simulink model "dsp_project"  (R2024b)
settings: Solver=VariableStepAuto  StartTime=0.0  StopTime=50  RelTol=1e-3
values from neighbouring files (symbols this model uses):
  Lf = max(1, round(freq_mask_smooth_hz / (fs/nfft)))    [dsp_project_matalb.m]    (also in dsp_project_nonstaion.m)
  Lt = max(1, round(time_mask_smooth_ms / (hop/fs*1e3)))    [dsp_project_matalb.m]    (also in dsp_project_nonstaion.m)
  n_std_thresh = 1.2    [dsp_project_matalb.m]    (also in dsp_project_nonstaion.m = 1.5)
libraries: dspvision x3, dspxfrm3 x2, dspstat3 x2, dspsigops x1
settings Model: Creator=settlab  LastModifiedBy=settlab

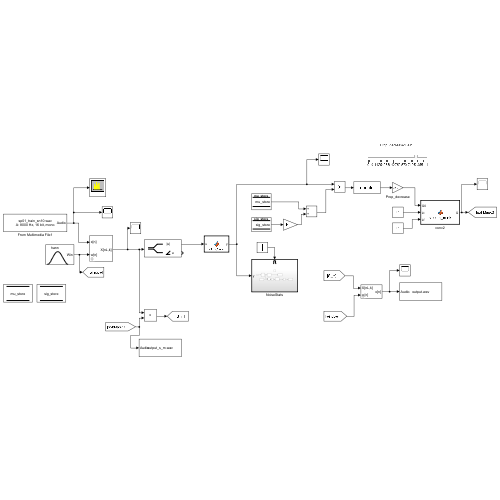
[thumbnail: Simulink's stored preview of the top-level diagram]
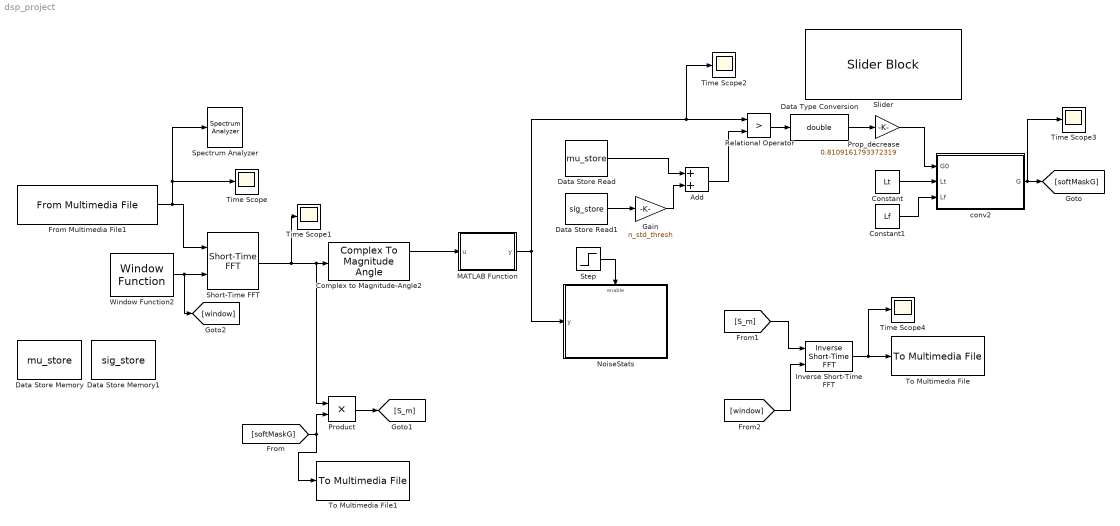
== system dsp_project ==
  Add : Sum
  Complex to Magnitude-Angle2 : ComplexToMagnitudeAngle
  Constant : Constant  Value=Lt
  Constant1 : Constant  Value=Lf
  Data Store Memory : DataStoreMemory  DataStoreName=mu_store  WriteAfterWriteMsg=warning  InitialValue=zeros(1024,1)  VectorParams1D=off  ShowAdditionalParam=off  OutDataTypeStr=double
  Data Store Memory1 : DataStoreMemory  DataStoreName=sig_store  WriteAfterWriteMsg=warning  InitialValue=zeros(1024,1)  VectorParams1D=off  ShowAdditionalParam=off  OutDataTypeStr=double
  Data Store Read : DataStoreRead  DataStoreName=mu_store  DataStoreElements=mu_store  EnableIndexing=on  NumberOfDimensions=2  IndexOptions=Index vector (dialog),Index vector (dialog)  Indices=1,1  OutputSizes=1,1
  Data Store Read1 : DataStoreRead  DataStoreName=sig_store  DataStoreElements=sig_store  EnableIndexing=on  NumberOfDimensions=2  IndexOptions=Index vector (dialog),Index vector (dialog)  Indices=1,1  OutputSizes=1,1
  Data Type Conversion : DataTypeConversion  OutDataTypeStr=double  SaturateOnIntegerOverflow=off  RndMeth=Floor
  From Multimedia File1 : dspvision/From Multimedia File  inputFilename=C:\Users\settlab\Downloads\sp01_train_sn10.wav  readRange=[1 Inf]  loop=on  numPlays=inf  outputStreams=오디오 전용  videoDataType=single  audioDataType=double  inheritSampleTime=on  userDefinedSampleTime=fs  noAudioOutput=off  isIntensityVideo=off  fourcc=RGB  colorVideoFormat=One multidimensional signal  outputEOF=off  dataOrg=Column-major  audioFrameSize=1024  computeAudioFrameSize=off  outSamplingMode=Sample based
      settings: LibrarySourceBlock=dspsrcs4/From Multimedia File
  Gain : Gain  Gain=n_std_thresh
  Inverse Short-Time FFT : dspxfrm3/Inverse  Short-Time FFT  W=1024  OvLap=768  OutFrameSize=256  InConjSymm=on  DoAssert=on  Tol=1e-4  OutputFrames=off
  MATLAB Function : MATLAB Function  TreatAsAtomicUnit=on
  NoiseStats : Subsystem  TreatAsAtomicUnit=on
  Product : Product
  Prop_decrease : Gain  Gain=0.8109161793372319  RndMeth=Nearest
  Relational Operator : RelationalOperator  Operator=>  OutDataTypeStr=boolean  ZeroCross=off  InputSameDT=off
  Short-Time FFT : dspxfrm3/Short-Time FFT  W=1024  OvLap=768  M=1024
  Slider : SliderBlock  ScaleMax=1
  Spectrum Analyzer : SpectrumAnalyzer  WindowPosition=[371.000000,449.000000,800.000000,572.000000,]  Visible=on  ScopeFrameLocation=window  ViewType=Spectrum and spectrogram  Method=Welch  PlotAsTwoSidedSpectrum=off  AveragingMethod=Exponential  YLimits=[-106.52525462,-0.29681245]  ColorLimits=[-106.52525462,-0.29681245]
  Step : Step  Time=0.5  Before=1  After=0  VectorParams1D=off  ZeroCross=off
  Time Scope{,1..4} (5 alike) : Scope
  To Multimedia File : dspvision/To Multimedia File  outputFilename=C:\Users\settlab\Documents\MATLAB\EIS_SSG\output.wav  streamSelection=Audio only  videoCompressor=None (uncompressed)  audioCompressor=None (uncompressed)  imagePorts=One multidimensional signal  fileType=WAV  audioDatatype=16-bit integer  fourcc=RGB  audioBitRate=128  audioQuality=75  videoQuality=75  mj2000CompFactor=10
      settings: LibrarySourceBlock=dspsnks4/To Multimedia File
  To Multimedia File1 : dspvision/To Multimedia File  outputFilename=C:\Users\settlab\Documents\MATLAB\EIS_SSG\output_s_m.wav  streamSelection=Audio only  videoCompressor=None (uncompressed)  audioCompressor=None (uncompressed)  imagePorts=One multidimensional signal  fileType=WAV  audioDatatype=16-bit integer  fourcc=RGB  audioBitRate=128  audioQuality=75  videoQuality=75  mj2000CompFactor=10
      settings: LibrarySourceBlock=dspsnks4/To Multimedia File
  Window Function2 : dspsigops/Window Function  winmode=Generate window  wintype=Hann  sampmode=Discrete  samptime=-1  N=1024  Rs=50  beta=10  winsamp=Symmetric  UserWindow=hamming  OptParams=off  UserParams={'symmetric'}  dataType=double  isSigned=on  wordLen=16  udDataType=sfix(16)  fracBitsMode=Best precision  numFracBits=15  roundingMode=Floor  overflowMode=off  numSidelobes=4  sidelobeLevel=-30
  conv2 : MATLAB Function  TreatAsAtomicUnit=on
  wires:
  From Multimedia File1/1 -> Spectrum Analyzer/1, Time Scope/1, Short-Time FFT/1
  Complex to Magnitude-Angle2/1 -> MATLAB Function/1(u)
  MATLAB Function/1(y) -> NoiseStats/1(y), Time Scope2/1, Relational Operator/1
  Step/1 -> NoiseStats/Enable
  Data Store Read1/1 -> Gain/1
  Data Store Read/1 -> Add/1
  Gain/1 -> Add/2
  Add/1 -> Relational Operator/2
  Relational Operator/1 -> Data Type Conversion/1
  Data Type Conversion/1 -> Prop_decrease/1
  Prop_decrease/1 -> conv2/1(G0)
  Short-Time FFT/1 -> Time Scope1/1, Product/1, Complex to Magnitude-Angle2/1
  [softMaskG] -> Product/2, To Multimedia File1/1
  Product/1 -> [S_m]
  [S_m] -> Inverse Short-Time FFT/1
  Window Function2/1 -> [window], Short-Time FFT/2
  [window] -> Inverse Short-Time FFT/2
  Inverse Short-Time FFT/1 -> Time Scope4/1, To Multimedia File/1
  Constant/1 -> conv2/2(Lt)
  Constant1/1 -> conv2/3(Lf)
  conv2/1(G) -> Time Scope3/1, [softMaskG]

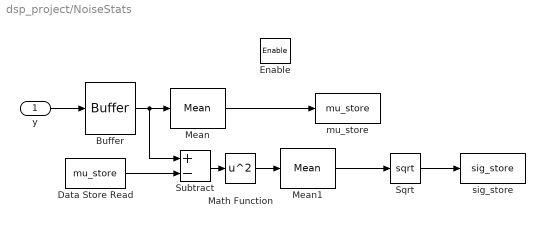
== system dsp_project/NoiseStats ==
  y : Inport
  Enable : EnablePort
  Buffer : Buffer  N=1024  V=1  OutputFrames=off
  Data Store Read : DataStoreRead  DataStoreName=mu_store  IndexOptions=Index vector (dialog)  Indices=1  OutputSizes=1
  Math Function : Math  Operator=square
  Mean : dspstat3/Mean  run=on  reset_popup=None  directionMode=Each row  dimension=1  roiEnable=off  roiType=Rectangles  roiPortion=Entire ROI  roiOutput=Individual statistics for each ROI  roiFlag=off  roundingMode=Floor  overflowMode=off  outputDataTypeStr=Inherit: Same as accumulator  outputMin=[]  outputMax=[]  outputLastDataTypeStr=Inherit: Same as accumulator
  Mean1 : dspstat3/Mean  run=on  reset_popup=None  directionMode=Each row  dimension=1  roiEnable=off  roiType=Rectangles  roiPortion=Entire ROI  roiOutput=Individual statistics for each ROI  roiFlag=off  roundingMode=Floor  overflowMode=off  outputDataTypeStr=Inherit: Same as accumulator  outputMin=[]  outputMax=[]  outputLastDataTypeStr=Inherit: Same as accumulator
  Sqrt : Sqrt  OutputSignalType=real  SaturateOnIntegerOverflow=off
  Subtract : Sum  Inputs=+-
  mu_store : DataStoreWrite  DataStoreName=mu_store  DataStoreElements=mu_store  NumberOfDimensions=2  IndexOptions=Index vector (dialog),Index vector (dialog)  Indices=1,1  OutputSizes=1,1
  sig_store : DataStoreWrite  DataStoreName=sig_store  DataStoreElements=sig_store  NumberOfDimensions=2  IndexOptions=Index vector (dialog),Index vector (dialog)  Indices=1,1  OutputSizes=1,1
  wires:
  Buffer/1 -> Subtract/1, Mean/1
  Mean/1 -> mu_store/1
  y/1 -> Buffer/1
  Sqrt/1 -> sig_store/1
  Mean1/1 -> Sqrt/1
  Data Store Read/1 -> Subtract/2
  Subtract/1 -> Math Function/1
  Math Function/1 -> Mean1/1

== matlab function dsp_project/MATLAB Function ==
  data: u input; y output
function y = db_Conv(u)
y = 20*log10(u + eps);
end

== matlab function dsp_project/conv2 ==
  data: G0 input; G output; Lt input; Lf input
function G = smooth_mask(G0, Lt, Lf)
%#codegen
% G0 : soft mask (double matrix) [freqBins x timeFrames]
% Lt, Lf : kernel 길이

% 1D 삼각 커널
kt = triang(Lt); kf = triang(Lf);
K2D = (kt* kf.') / sum(kt)*sum(kf);   % 정규화

% 2-D convolution (same size)
G = conv2(G0, K2D, 'same');
end
